simulink model "pwm_rectifier"  (Simulink 6.1)
settings: Solver=ode23tb  StartTime=0.0  StopTime=0.0799  MaxStep=5e-6  RelTol=1e-3  AbsTol=.01
libraries: powerlib x9, simulink x1
settings Model: LastModifiedBy=ThinkPad
settings DebuggingCC: SolverPrmCheckMsg=warning

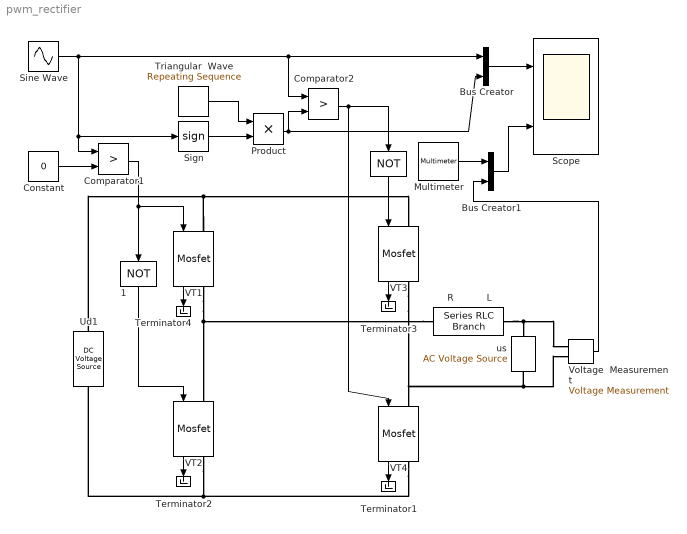
== system pwm_rectifier ==
  " " : Logic  Orientation=down  Operator=NOT  AllPortsSameDT=off  OutDataTypeMode=Boolean
  " 1" : Logic  Orientation=down  Operator=NOT  AllPortsSameDT=off  OutDataTypeMode=Boolean
  Bus Creator : BusCreator  DialogController=Simulink.DDGSource_Bus  Inputs=2
  Bus Creator1 : BusCreator  DialogController=Simulink.DDGSource_Bus  Inputs=2
  Comparator1 : RelationalOperator  Operator=>  LogicOutDataTypeMode=Boolean  LogicDataType=sint(32)  ZeroCross=off
  Comparator2 : RelationalOperator  Operator=>  LogicOutDataTypeMode=Boolean  LogicDataType=sint(32)  ZeroCross=off
  Constant : Constant  Value=0
  Multimeter : powerlib/Measurements/Multimeter  PhasorSimulation=off  OutputType=Complex  sel=2  L=2  Gain=1  yselected="{'Ib: R           L'};"  PSBOutputType=1  PSBequivalent=0  AxesSetting=[0,0.1,-100,100]  Display=0  SavedBlockNames=-11
  Product : Product  RndMeth=Zero
  R           L : powerlib/Elements/Series RLC Branch  PhysicalDomain=powersysdomain  SubClassName=unknown  LeftPortType=p1  RightPortType=p1  LConnTagsString=__new0  RConnTagsString=__new0  Resistance=0.5  Inductance=0.01  Capacitance=inf  Measurements=Branch voltage and current
  Scope : Scope  NumInputPorts=2
      settings: TimeRange=0.04  YMin=-1.5~-50  YMax=1.5~50  SampleTime=2e-4
  Sign : Signum
  Sine Wave : Sin  Amplitude=0.8  Frequency=314  SampleTime=0
  Terminator{1..4} (4 alike) : Terminator
      settings: Orientation=down
  Triangular  Wave : simulink/Sources/Repeating Sequence  rep_seq_t=[0 5e-4 1e-3]  rep_seq_y=[1 0 1]
  Ud1 : powerlib/Electrical Sources/DC Voltage Source  Orientation=up  Amplitude=100  Measurements=None
  VT{1..4} (4 alike) : powerlib/Power Electronics/Mosfet  Orientation=down  Ron=0.01  Lon=1e-7  Rd=.01  IC=0  Rs=5  Cs=1e-6  Measurements=on
  Voltage  Measurement : powerlib/Measurements/Voltage Measurement  PhasorSimulation=off  OutputType=Complex  PSBequivalent=0
  us : powerlib/Electrical Sources/AC Voltage Source  Orientation=up  Amplitude=50  Phase=-45  Frequency=50  SampleTime=0  Measurements=None
  wires:
  Comparator2/1 -> " "/1, VT4/1
  VT4/1 -> Terminator1/1
  VT2/1 -> Terminator2/1
  VT3/1 -> Terminator3/1
  Sine Wave/1 -> Sign/1, Comparator1/1, Bus Creator/1, Comparator2/1
  Bus Creator/1 -> Scope/1
  " "/1 -> VT3/1
  VT1/1 -> Terminator4/1
  Sign/1 -> Product/2
  " 1"/1 -> VT2/1
  Triangular  Wave/1 -> Product/1
  Product/1 -> Comparator2/2, Bus Creator/2
  Comparator1/1 -> VT1/1, " 1"/1
  Constant/1 -> Comparator1/2
  Multimeter/1 -> Bus Creator1/1
  Voltage  Measurement/1 -> Bus Creator1/2
  Bus Creator1/1 -> Scope/2
  connections:
  VT3/RConn1 -- VT4/LConn1 -- us/LConn1 -- Voltage  Measurement/LConn2
  VT1/RConn1 -- VT2/LConn1 -- R           L/LConn1
  VT4/RConn1 -- Ud1/LConn1 -- VT2/RConn1
  VT1/LConn1 -- VT3/LConn1 -- Ud1/RConn1
  R           L/RConn1 -- us/RConn1 -- Voltage  Measurement/LConn1
